simulink model "tsat_ol_original"  (Simulink 6.6)
settings: Solver=FixedStepDiscrete  SolverMode=SingleTasking  StartTime=0.0  StopTime=3  FixedStep=.1  RelTol=1e-3
libraries: simulink x2
settings Model: Creator=rob  LastModifiedBy=Administrator  ExtModeAutoUpdateStatusClock=off
settings DataIOCC: SignalLoggingName=sigsOut
settings OptimizationCC: InlineInvariantSignals=on
settings DebuggingCC: SignalResolutionControl=TryResolveAllWithWarning  SolverPrmCheckMsg=none  MultiTaskDSMMsg=warning  MultiTaskCondExecSysMsg=none  StrictBusMsg=None
settings HardwareCC: TargetUnknown=on
settings RTWCC: IncludeERTFirstTime=on

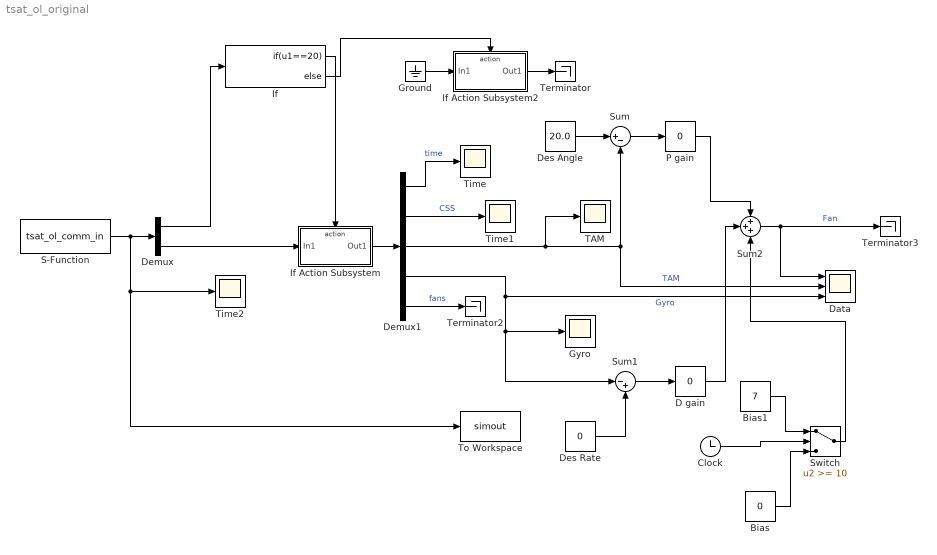
== system tsat_ol_original ==
  Bias : Constant  Value=0
  Bias1 : Constant  Value=7
  Clock : Clock
      settings: Decimation=10
  D gain : simulink/Math Operations/Slider Gain  SystemSampleTime=-1  low=-15  gain=0  high=20
  Data : Scope  NumInputPorts=3
      settings: TimeRange=100  YMin=0~-200~-35  YMax=7~200~5
  Demux : Demux  Outputs=[1;-1]
  Demux1 : Demux  Outputs=[1;11;1;1;2]
  Des Angle : Constant  Value=20.0  OutDataTypeMode=double
  Des Rate : Constant  Value=0  OutDataTypeMode=double
  Ground : Ground
  Gyro : Scope
      settings: TimeRange=100  YMin=9.65  YMax=10.45  SaveName=GyroData
  If : If  IfExpression=u1==20
  If Action Subsystem : Subsystem  TreatAsAtomicUnit=on
  If Action Subsystem2 : Subsystem  TreatAsAtomicUnit=on
  P gain : simulink/Math Operations/Slider Gain  SystemSampleTime=-1  low=-15  gain=0  high=30
  S-Function : S-Function  FunctionName=tsat_ol_comm_in
  Sum : Sum  Inputs=|+-  SaturateOnIntegerOverflow=on
  Sum1 : Sum  Inputs=|-+  SaturateOnIntegerOverflow=on
  Sum2 : Sum  Inputs=+++  SaturateOnIntegerOverflow=on
  Switch : Switch  Threshold=10
  TAM : Scope
      settings: TimeRange=100  YMin=5  YMax=35  SaveName=TAMData
  Terminator : Terminator
  Terminator2 : Terminator
  Terminator3 : Terminator
  Time : Scope
      settings: TimeRange=100  YMin=-1  YMax=1  SaveName=TimeData
  Time1 : Scope
      settings: TimeRange=100  YMin=-175  YMax=200  SaveName=TimeData1
  Time2 : Scope
      settings: TimeRange=100  YMin=-1  YMax=1  SaveName=TimeData2
  To Workspace : ToWorkspace  VariableName=simout  SampleTime=-1  SaveFormat=Array
  wires:
  If/1 -> If Action Subsystem/Action
  If/2 -> If Action Subsystem2/Action
  Demux/1 -> If/1
  S-Function/1 -> Demux/1, Time2/1, To Workspace/1
  If Action Subsystem2/1(Out1) -> Terminator/1
  Demux/2 -> If Action Subsystem/1(In1)
  Ground/1 -> If Action Subsystem2/1(In1)
  If Action Subsystem/1(Out1) -> Demux1/1
  Des Angle/1 -> Sum/1
  Des Rate/1 -> Sum1/2
  Sum1/1 -> D gain/1
  Sum/1 -> P gain/1
  P gain/1 -> Sum2/1
  D gain/1 -> Sum2/2
  Sum2/1 -> Data/1, Terminator3/1  "Fan"
  Demux1/5 -> Terminator2/1  "fans"
  Demux1/1 -> Time/1  "time"
  Demux1/2 -> Time1/1  "CSS"
  Demux1/3 -> Sum/2, Data/2, TAM/1  "TAM"
  Demux1/4 -> Data/3, Sum1/1, Gyro/1  "Gyro"
  Bias1/1 -> Switch/1
  Bias/1 -> Switch/3
  Clock/1 -> Switch/2
  Switch/1 -> Sum2/3

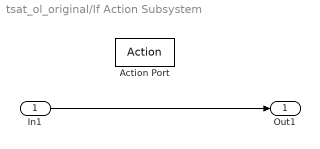
== system tsat_ol_original/If Action Subsystem ==
  In1 : Inport
  Action Port : ActionPort  ActionType=then
  Out1 : Outport
  wires:
  In1/1 -> Out1/1

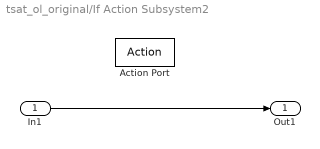
== system tsat_ol_original/If Action Subsystem2 ==
  In1 : Inport
  Action Port : ActionPort  ActionType=else
  Out1 : Outport
  wires:
  In1/1 -> Out1/1
